simulink model "environment_simulation"  (R2022a)
settings: Solver=ode15s  StartTime=0.0  StopTime=42000  RelTol=1e-3
InitFcn:
  | global LOData LOModelData gprMdlLP_machine1 gprMdlLP_machine2 gprMdlLP_machine3 gprMdlLP_machine4 gprMdlLP_machine5 significance SteadyState explore explore_signal
  | load load_opt_multiple_init.mat
undefined symbols (not defined in the file or in its folder): sigbuilder_block
libraries: slpidlib x12, simulink x10
(part 1 of 2)
settings Model: Creator=Memo Mer  LastModifiedBy=busesibelkorkmaz
settings SolverCC: AlgebraicLoopSolver=TrustRegion
settings DebuggingCC: UnconnectedInputMsg=warning  UnconnectedOutputMsg=warning  UnconnectedLineMsg=warning  SFMachineParentedDataDiag=warning
settings RTWCC: DLArmComputeVersion=19.05

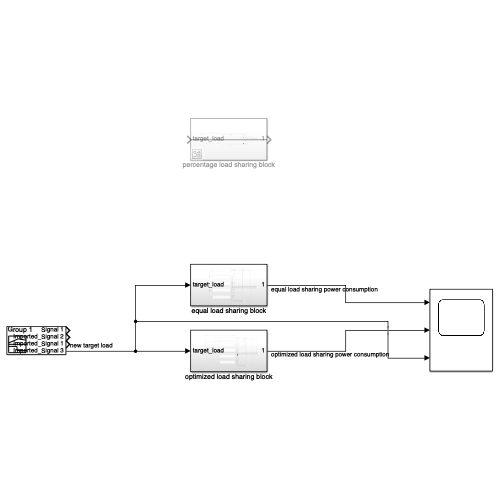
[thumbnail: Simulink's stored preview of the top-level diagram]
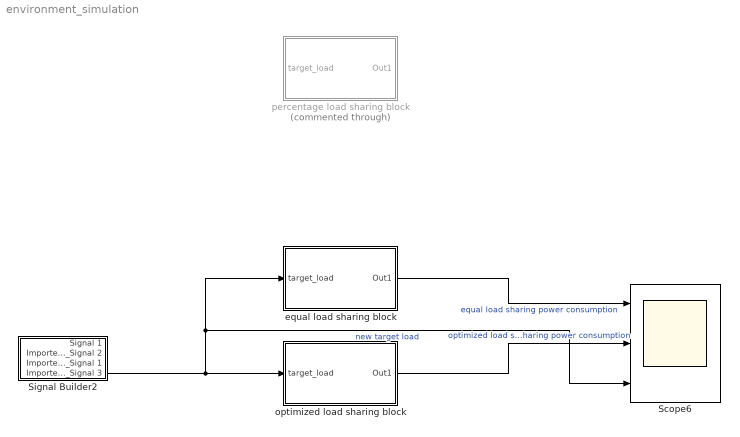
== system environment_simulation ==
  Scope6 : Scope  NumInputPorts=3
  Signal Builder2 : Subsystem  Tag=STV Subsys  LoadFcn=sigbuilder_block('load');  StartFcn=sigbuilder_block('start');  StopFcn=sigbuilder_block('stop');  ClipboardFcn=sigbuilder_block('clipboard');  mask(Sigbuilder block){tuvar=[0:10]}
      mask help: Simulink:masks:SigbuilderBlock_MD
      mask init:
      | if ~strcmp(get_param(bdroot(gcbh),'SimulationStatus'),'stopped') tuvar = sigbuilder_block('maskInit'); end
      settings: CopyFcn=sigbuilder_block('copy');  DeleteFcn=sigbuilder_block('delete');  ModelCloseFcn=sigbuilder_block('modelClose');  PreSaveFcn=sigbuilder_block('preSave');  PauseFcn=sigbuilder_block('pause');  ContinueFcn=sigbuilder_block('continue');  NameChangeFcn=sigbuilder_block('namechange');  OpenFcn=sigbuilder_block('open',[13 58 890 740 ]);  CloseFcn=sigbuilder_block('close');
      mask Display: plot(0, 0, 100, 100,[2, 2, 32, 32, 2], [68, 8, 8, 68, 68],[32, 2], [38, 38], [32, 19, 2],[53, 60, 44], [32, 17, 17, 2],[16, 16, 31, 31]);txt = getActiveGroup(gcbh);text(2, 100, txt,'verticalAlignment', 'top');
  equal load sharing block : Subsystem  Tag=equal load sharing
  optimized load sharing block : Subsystem  Tag=equal load sharing
  percentage load sharing block : Subsystem  Tag=equal load sharing  Commented=through
  wires:
  Signal Builder2/4(Imported_Signal 3) -> Scope6/3, equal load sharing block/1(target_load), optimized load sharing block/1(target_load)  "new target load"
  optimized load sharing block/1(Out1) -> Scope6/2  "optimized load sharing power consumption"
  equal load sharing block/1(Out1) -> Scope6/1  "equal load sharing power consumption"

== system environment_simulation/Signal Builder2 ==
  Demux : Demux  Tag=STV Demux
      settings: DisplayOption=none
  FromWs : FromWorkspace  Tag=STV FromWs  VariableName=tuvar
      SigBuilderData=|
      | common.afterFinalStr = 'Extrapolate'
      | common.sampleTime = '0'
      | dataSet.timeRange = [0 42000]
      | dataSet.name = 'Group 1'
      | sbobj.Groups.Name = 'Group 1'
      | sbobj.Groups.Signals(1).Name = 'Signal 1'
      | sbobj.Groups.Signals(1).XData = [0 200 200 400 400 600 600 800 800 1000 1000 1200 1200 1400 1400 1600 1600 1800 1800 2000 2000 2200 2200 2400 2400 2600 2620 4200 42000]
      | sbobj.Groups.Signals(1).YData = [0 0 -3.904416471 -3.904416471 -9.753929308 -9.753929308 -21.01201906 -21.01201906 -32.66837352 -32.66837352 3.755067207 3.755067207 7.595476851 7.5955 23.08157315 23.0816 19.1700448 19.1700448 28.04921414 28.04921414 27.99587512 27.99587512 28.33368893 28.3337 20.90889695 20.90889695 28.67505867 28.5998696218 28.5998696218]
      | sbobj.Groups.Signals(2).Name = 'Imported_Signal 2'
      | sbobj.Groups.Signals(2).XData = [0 200 200 400 400 600 600 800 800 1000 1000 1200 1200 1400 1400 1600 1600 1800 1800 2000 2000 2200 2200 2400 2400 2600 2600 2800 2800 3000 3000 3200 3200 3400 3400 3600 3600 3800 3800 4000 4000 42000]
      | sbobj.Groups.Signals(2).YData = [67.81523362 67.81523362 63.91081715 63.91081715 58.06130431 58.06130431 46.80321456 46.80321456 35.1468601 35.1468601 71.57030083 71.57030083 75.41071047 75.41071047 90.89680677 90.89680677 86.98527842 86.98527842 95.86444776 95.86444776 95.81110874 95.81110874 96.14892255 96.14892255 96.49029229 96.49029229 88.72413057 88.72413057 75.49249697 75.49249697 54.52670507 54.52670507 32.00341369 32.00341369 38.94815446 38.94815446 22.26370812 22.26370812 22.9855629 22.9855629 11.35409999 11.35409999]
      | sbobj.Groups.Signals(3).Name = 'Imported_Signal 1'
      | sbobj.Groups.Signals(3).XData = [0 200 200 400 400 600 600 800 800 1000 1000 1200 1200 1400 1400 1600 1600 1800 1800 2000 2000 2200 2200 2400 2400 2600 2600 2800 2800 3000 3000 3200 3200 3400 3400 3600 3600 3800 3800 4000 4000 42000]
      | sbobj.Groups.Signals(3).YData = [2130.75464 2130.75464 2008.077875 2008.077875 1824.286181 1824.286181 1470.557001 1470.557001 1104.314344 1104.314344 2248.738852 2248.738852 2369.404523 2369.404523 2855.977669 2855.977669 2733.077448 2733.077448 3012.060949 3012.060949 3010.385037 3010.385037 3020.999147 3020.999147 3031.724984 3031.724984 2787.712183 2787.712183 2371.974255 2371.974255 1713.229073 1713.229073 1005.547258 1005.547258 1223.751013 1223.751013 699.5257091 699.5257091 722.2063863 722.2063863 356.7458217 356.7458217]
      | sbobj.Groups.Signals(4).Name = 'Imported_Signal 3'
      | sbobj.Groups.Signals(4).XData = [0 1000 1000 2000 2000 3000 3000 4000 4000 5000 5000 6000 6000 7000 7000 8000 8000 9000 9000 10000 10000 11000 11000 12000 12000 13000 13000 14000 14000 15000 15000 16000 16000 17000 17000 18000 18000 19000 19000 20000 20000 21000 21000 22000 22000 23000 23000 24000 24000 25000 25000 26000 26000 27000 27000 28000 28000 29000 29000 30000 30000 31000 31000 32000 32000 33000 33000 34000 34000 35000 35000 36000 36000 37000 37000 38000 38000 39000 39000 40000 40000 41000 41000 42000]
      | sbobj.Groups.Signals(4).YData = [2130.75464 2130.75464 2008.077875 2008.077875 1824.286181 1824.286181 1470.557001 1470.557001 1104.314344 1104.314344 2248.738852 2248.738852 2369.404523 2369.404523 2855.977669 2855.977669 2733.077448 2733.077448 3012.060949 3012.060949 3010.385037 3010.385037 3020.999147 3020.999147 3031.724984 3031.724984 2787.712183 2787.712183 2371.974255 2371.974255 1713.229073 1713.229073 1005.547258 1005.547258 1223.751013 1223.751013 699.5257091 699.5257091 722.2063863 722.2063863 356.7458217 356.7458217 391.7165208 391.7165208 658.6334542 658.6334542 292.2790697 292.2790697 132.7322379 132.7322379 473.2775761 473.2775761 240.7727045 240.7727045 654.2760827 654.2760827 1287.435673 1287.435673 1396.258232 1396.258232 2089.862385 2089.862385 1516.812175 1516.812175 2198.573217 2198.573217 1028.8983 1028.8983 2684.81118 2684.81118 601.7641704 601.7641704 2757.210582 2757.210582 2915.081502 2915.081502 2281.363274 2281.363274 1670.549178 1670.549178 1876.909821 1876.909821 1425.53083 1425.53083]
      | sbobj.Groups.TimeRange = [0 42000]
  Signal 1 : Outport  Tag=STV Outport
  Imported_Signal 2 : Outport  Tag=STV Outport  Port=2
  Imported_Signal 1 : Outport  Tag=STV Outport  Port=3
  Imported_Signal 3 : Outport  Tag=STV Outport  Port=4
  wires:
  Demux/1 -> Signal 1/1
  FromWs/1 -> Demux/1
  Demux/2 -> Imported_Signal 2/1
  Demux/3 -> Imported_Signal 1/1
  Demux/4 -> Imported_Signal 3/1

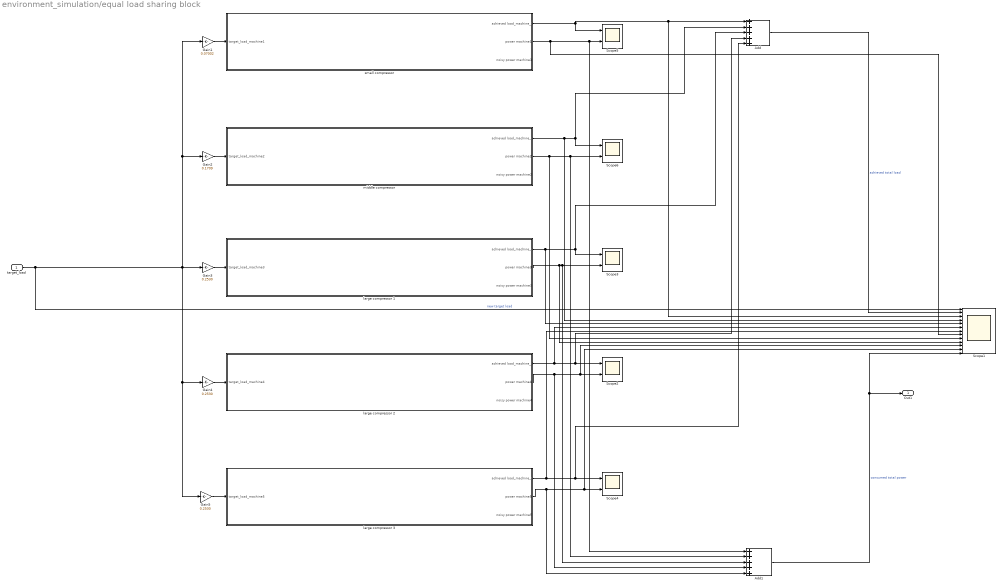
== system environment_simulation/equal load sharing block ==
  target_load : Inport
  Add : Sum  Inputs=+++++
  Add1 : Sum  Inputs=+++++
  Gain1 : Gain  Gain=0.07002
  Gain2 : Gain  Gain=0.1709
  Gain3 : Gain  Gain=0.2530
  Gain4 : Gain  Gain=0.2530
  Gain5 : Gain  Gain=0.2530
  Scope1 : Scope  NumInputPorts=13
  Scope{2..6} (5 alike) : Scope  NumInputPorts=2
  large compressor 1 : Subsystem
  large compressor 2 : Subsystem
  large compressor 3 : Subsystem
  middle compressor : Subsystem
  small compressor : Subsystem
  Out1 : Outport
  wires:
  Add/1 -> Scope1/2  "achieved total load"
  large compressor 1/1(achieved load_machine_3) -> Scope1/5, Scope3/1, Add/3
  middle compressor/1(achieved load_machine_2) -> Scope1/4, Scope6/1, Add/2
  small compressor/2(power machine1) -> Scope1/8, Add1/1, Scope5/2
  large compressor 3/1(achieved load_machine_5) -> Scope1/7, Add/5, Scope4/1
  middle compressor/2(power machine2) -> Scope1/9, Add1/2, Scope6/2
  large compressor 3/2(power machine5) -> Add1/5, Scope1/12, Scope4/2
  large compressor 2/2(power machine4) -> Add1/4, Scope1/11, Scope2/2
  target_load/1 -> Gain1/1, Gain2/1, Gain5/1, Gain4/1, Gain3/1, Scope1/1  "new target load"
  small compressor/1(achieved load_machine_1) -> Scope5/1, Scope1/3, Add/1
  Add1/1 -> Out1/1, Scope1/13  "consumed total power"
  large compressor 1/2(power machine3) -> Scope1/10, Add1/3, Scope3/2
  large compressor 2/1(achieved load_machine_4) -> Scope1/6, Add/4, Scope2/1
  Gain1/1 -> small compressor/1(target_load_machine1)
  Gain2/1 -> middle compressor/1(target_load_machine2)
  Gain3/1 -> large compressor 1/1(target_load_machine3)
  Gain4/1 -> large compressor 2/1(target_load_machine4)
  Gain5/1 -> large compressor 3/1(target_load_machine5)

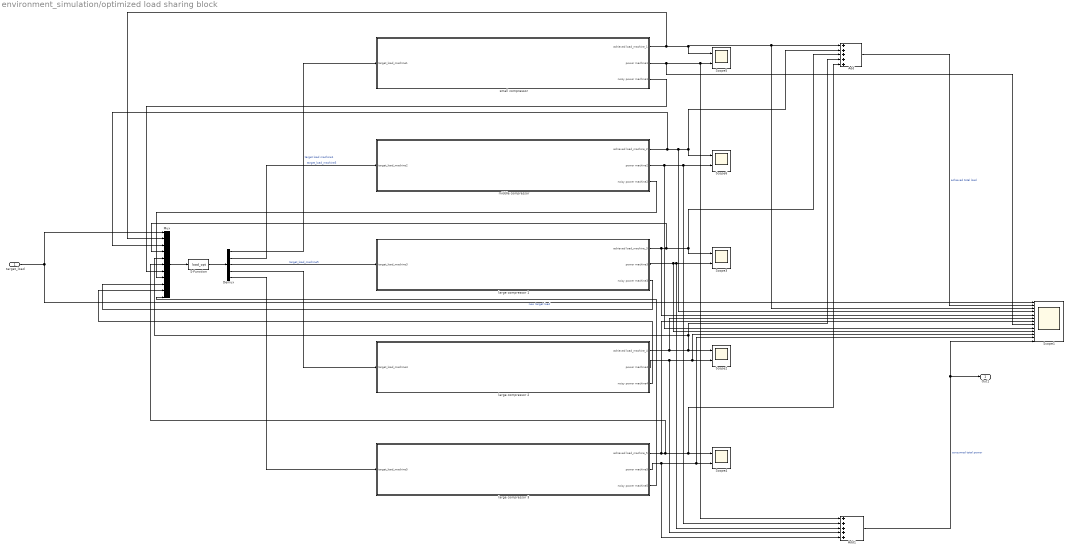
== system environment_simulation/optimized load sharing block ==
  target_load : Inport
  Add : Sum  Inputs=+++++
  Add1 : Sum  Inputs=+++++
  Demux : Demux  Outputs=5
  Mux : Mux  Inputs=11
  S-Function : S-Function  FunctionName=load_opt  Parameters=[],[]  SFunctionDeploymentMode=off  EnableBusSupport=off
  Scope1 : Scope  NumInputPorts=13
  Scope{2..6} (5 alike) : Scope  NumInputPorts=2
  large compressor 1 : Subsystem
  large compressor 2 : Subsystem
  large compressor 3 : Subsystem
  middle compressor : Subsystem
  small compressor : Subsystem
  Out1 : Outport
  wires:
  Add/1 -> Scope1/2  "achieved total load"
  Add1/1 -> Out1/1, Scope1/13  "consumed total power"
  Mux/1 -> S-Function/1
  target_load/1 -> Mux/1, Scope1/1  "new target load"
  S-Function/1 -> Demux/1
  large compressor 1/1(achieved load_machine_3) -> Scope1/5, Mux/4, Scope3/1, Add/3
  large compressor 3/1(achieved load_machine_5) -> Scope1/7, Mux/6, Add/5, Scope4/1
  large compressor 3/2(power machine5) -> Add1/5, Scope1/12, Scope4/2
  middle compressor/1(achieved load_machine_2) -> Scope1/4, Scope6/1, Add/2, Mux/3
  middle compressor/2(power machine2) -> Scope1/9, Add1/2, Scope6/2
  small compressor/2(power machine1) -> Scope1/8, Add1/1, Scope5/2
  Demux/1 -> small compressor/1(target_load_machine1)  "target load machine1"
  Demux/2 -> middle compressor/1(target_load_machine2)  "target_load_machine5"
  Demux/3 -> large compressor 1/1(target_load_machine3)  "target_load_machine5"
  Demux/4 -> large compressor 2/1(target_load_machine4)
  Demux/5 -> large compressor 3/1(target_load_machine5)
  large compressor 3/3(noisy power machine5) -> Mux/11
  large compressor 2/3(noisy power machine4) -> Mux/10
  middle compressor/3(noisy power machine2) -> Mux/8
  large compressor 1/3(noisy power machine3) -> Mux/9
  small compressor/3(noisy power machine1) -> Mux/7
  small compressor/1(achieved load_machine_1) -> Scope5/1, Scope1/3, Add/1, Mux/2
  large compressor 1/2(power machine3) -> Scope1/10, Add1/3, Scope3/2
  large compressor 2/1(achieved load_machine_4) -> Scope1/6, Add/4, Mux/5, Scope2/1
  large compressor 2/2(power machine4) -> Add1/4, Scope1/11, Scope2/2

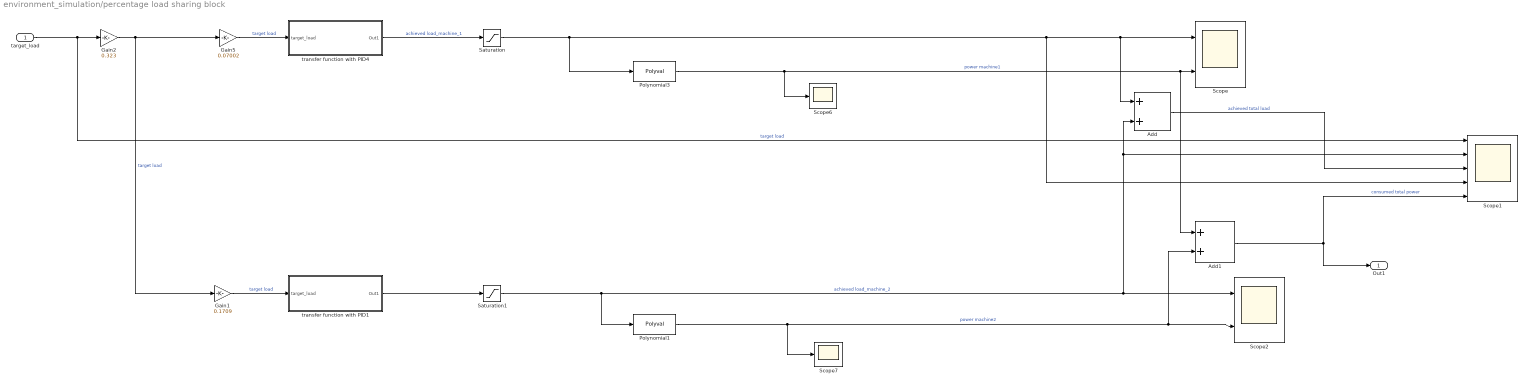
== system environment_simulation/percentage load sharing block ==
  target_load : Inport
  Add : Sum
  Add1 : Sum
  Gain1 : Gain  Gain=0.1709
  Gain2 : Gain  Gain=0.323
  Gain5 : Gain  Gain=0.07002
  Polynomial1 : Polyval  Coefs=[-1.42718017e-08 1.87477980e-05 -8.28649653e-03 1.88469092 -2.19952823]
  Polynomial3 : Polyval  Coefs=[-9e-08 4e-05 -0.0052 0.7765 15.661]
  Saturation : Saturate  UpperLimit=220  LowerLimit=56
  Saturation1 : Saturate  UpperLimit=537  LowerLimit=237
  Scope : Scope  NumInputPorts=2
  Scope1 : Scope  NumInputPorts=5
  Scope2 : Scope  NumInputPorts=2
  Scope6 : Scope
  Scope7 : Scope
  transfer function with PID1 : Subsystem
  transfer function with PID4 : Subsystem
  Out1 : Outport
  wires:
  Polynomial3/1 -> Scope6/1, Scope/2, Add1/1  "power machine1"
  transfer function with PID4/1(Out1) -> Saturation/1  "achieved load_machine_1"
  target_load/1 -> Gain2/1, Scope1/1  "target load"
  Saturation1/1 -> Polynomial1/1, Scope2/1, Add/2, Scope1/2  "achieved load_machine_2"
  transfer function with PID1/1(Out1) -> Saturation1/1
  Add/1 -> Scope1/3  "achieved total load"
  Add1/1 -> Scope1/5, Out1/1  "consumed total power"
  Polynomial1/1 -> Scope7/1, Scope2/2, Add1/2  "power machine2"
  Saturation/1 -> Polynomial3/1, Add/1, Scope/1, Scope1/4
  Gain5/1 -> transfer function with PID4/1(target_load)  "target load"
  Gain1/1 -> transfer function with PID1/1(target_load)  "target load"
  Gain2/1 -> Gain1/1, Gain5/1  "target load"

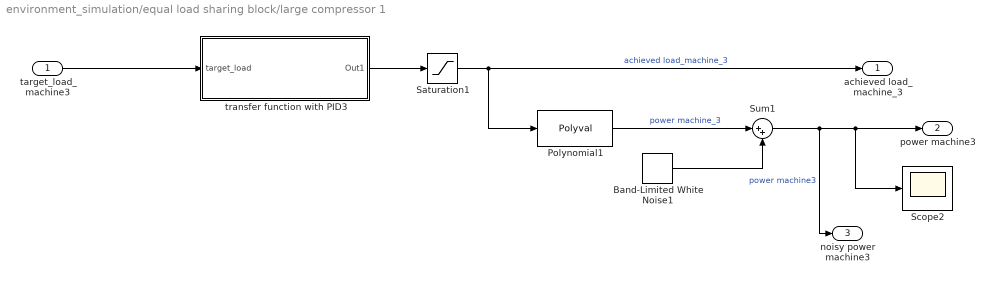
== system environment_simulation/equal load sharing block/large compressor 1 ==
  target_load_machine3 : Inport
  Band-Limited White Noise1 : simulink/Sources/Band-Limited White Noise  Cov=[0.1]  Ts=5  seed=[23341]
  Polynomial1 : Polyval  Coefs="[-1.53490519e-09  2.28838030e-06 -9.59520873e-04 6.18821903e-01 7.51758182e+01]"
  Saturation1 : Saturate  UpperLimit=795  LowerLimit=194
  Scope2 : Scope
  Sum1 : Sum  Inputs=|++
  transfer function with PID3 : Subsystem
  achieved load_machine_3 : Outport
  power machine3 : Outport  Port=2
  noisy power machine3 : Outport  Port=3
  wires:
  Polynomial1/1 -> Sum1/1  "power machine_3"
  target_load_machine3/1 -> transfer function with PID3/1(target_load)
  transfer function with PID3/1(Out1) -> Saturation1/1
  Band-Limited White Noise1/1 -> Sum1/2
  Saturation1/1 -> achieved load_machine_3/1, Polynomial1/1  "achieved load_machine_3"
  Sum1/1 -> noisy power machine3/1, power machine3/1, Scope2/1  "power machine3"

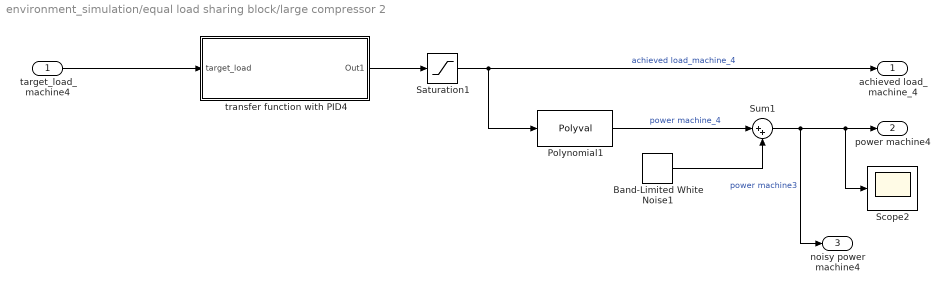
== system environment_simulation/equal load sharing block/large compressor 2 ==
  target_load_machine4 : Inport
  Band-Limited White Noise1 : simulink/Sources/Band-Limited White Noise  Cov=[0.1]  Ts=5  seed=[23341]
  Polynomial1 : Polyval  Coefs="[-1.53490519e-09  2.28838030e-06 -9.59520873e-04 6.18821903e-01 7.51758182e+01]"
  Saturation1 : Saturate  UpperLimit=795  LowerLimit=194
  Scope2 : Scope
  Sum1 : Sum  Inputs=|++
  transfer function with PID4 : Subsystem
  achieved load_machine_4 : Outport
  power machine4 : Outport  Port=2
  noisy power machine4 : Outport  Port=3
  wires:
  Polynomial1/1 -> Sum1/1  "power machine_4"
  Sum1/1 -> power machine4/1, Scope2/1, noisy power machine4/1  "power machine3"
  target_load_machine4/1 -> transfer function with PID4/1(target_load)
  transfer function with PID4/1(Out1) -> Saturation1/1
  Band-Limited White Noise1/1 -> Sum1/2
  Saturation1/1 -> achieved load_machine_4/1, Polynomial1/1  "achieved load_machine_4"

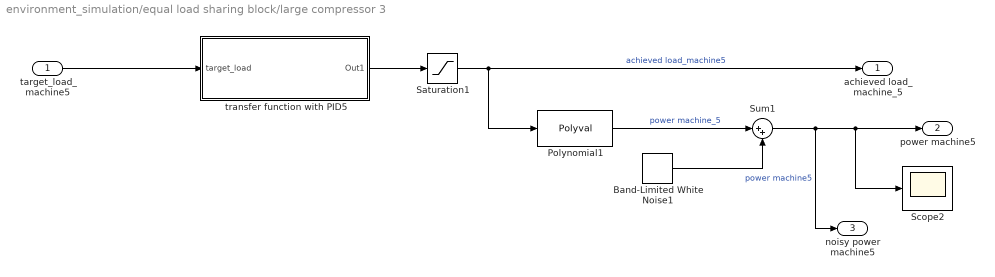
== system environment_simulation/equal load sharing block/large compressor 3 ==
  target_load_machine5 : Inport
  Band-Limited White Noise1 : simulink/Sources/Band-Limited White Noise  Cov=[0.1]  Ts=5  seed=[23341]
  Polynomial1 : Polyval  Coefs="[-1.53490519e-09  2.28838030e-06 -9.59520873e-04 6.18821903e-01 7.51758182e+01]"
  Saturation1 : Saturate  UpperLimit=795  LowerLimit=194
  Scope2 : Scope
  Sum1 : Sum  Inputs=|++
  transfer function with PID5 : Subsystem
  achieved load_machine_5 : Outport
  power machine5 : Outport  Port=2
  noisy power machine5 : Outport  Port=3
  wires:
  Polynomial1/1 -> Sum1/1  "power machine_5"
  target_load_machine5/1 -> transfer function with PID5/1(target_load)
  transfer function with PID5/1(Out1) -> Saturation1/1
  Band-Limited White Noise1/1 -> Sum1/2
  Saturation1/1 -> achieved load_machine_5/1, Polynomial1/1  "achieved load_machine5"
  Sum1/1 -> power machine5/1, Scope2/1, noisy power machine5/1  "power machine5"

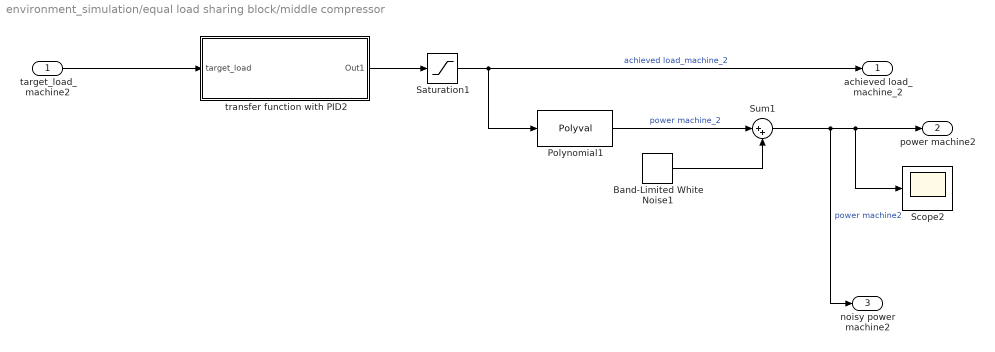
== system environment_simulation/equal load sharing block/middle compressor ==
  target_load_machine2 : Inport
  Band-Limited White Noise1 : simulink/Sources/Band-Limited White Noise  Cov=[0.1]  Ts=5  seed=[23341]
  Polynomial1 : Polyval  Coefs=[-1.42718017e-08 1.87477980e-05 -8.28649653e-03 1.88469092 -2.19952823]
  Saturation1 : Saturate  UpperLimit=537  LowerLimit=237
  Scope2 : Scope
  Sum1 : Sum  Inputs=|++
  transfer function with PID2 : Subsystem
  achieved load_machine_2 : Outport
  power machine2 : Outport  Port=2
  noisy power machine2 : Outport  Port=3
  wires:
  Polynomial1/1 -> Sum1/1  "power machine_2"
  target_load_machine2/1 -> transfer function with PID2/1(target_load)
  transfer function with PID2/1(Out1) -> Saturation1/1
  Band-Limited White Noise1/1 -> Sum1/2
  Saturation1/1 -> achieved load_machine_2/1, Polynomial1/1  "achieved load_machine_2"
  Sum1/1 -> noisy power machine2/1, power machine2/1, Scope2/1  "power machine2"

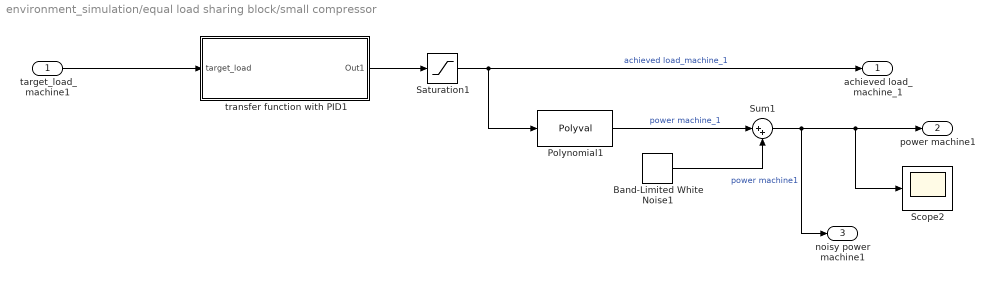
== system environment_simulation/equal load sharing block/small compressor ==
  target_load_machine1 : Inport
  Band-Limited White Noise1 : simulink/Sources/Band-Limited White Noise  Cov=[0.1]  Ts=5  seed=[23341]
  Polynomial1 : Polyval  Coefs=[-9e-08 4e-05 -0.0052 0.7765 15.661]
  Saturation1 : Saturate  UpperLimit=220  LowerLimit=56
  Scope2 : Scope
  Sum1 : Sum  Inputs=|++
  transfer function with PID1 : Subsystem
  achieved load_machine_1 : Outport
  power machine1 : Outport  Port=2
  noisy power machine1 : Outport  Port=3
  wires:
  Polynomial1/1 -> Sum1/1  "power machine_1"
  target_load_machine1/1 -> transfer function with PID1/1(target_load)
  transfer function with PID1/1(Out1) -> Saturation1/1
  Band-Limited White Noise1/1 -> Sum1/2
  Saturation1/1 -> achieved load_machine_1/1, Polynomial1/1  "achieved load_machine_1"
  Sum1/1 -> power machine1/1, Scope2/1, noisy power machine1/1  "power machine1"

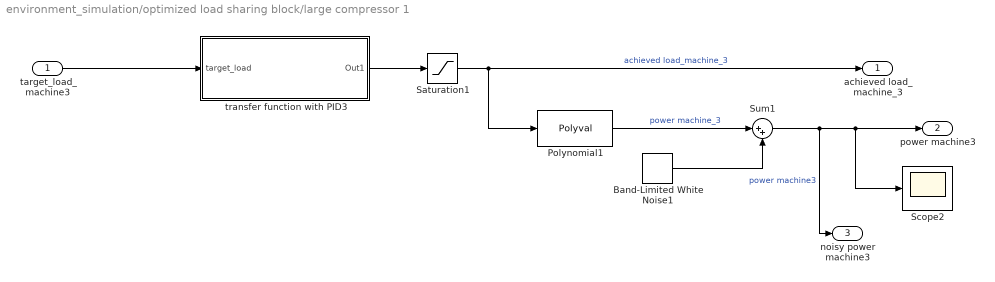
== system environment_simulation/optimized load sharing block/large compressor 1 ==
  target_load_machine3 : Inport
  Band-Limited White Noise1 : simulink/Sources/Band-Limited White Noise  Cov=[0.1]  Ts=5  seed=[23341]
  Polynomial1 : Polyval  Coefs="[-1.53490519e-09  2.28838030e-06 -9.59520873e-04 6.18821903e-01 7.51758182e+01]"
  Saturation1 : Saturate  UpperLimit=795  LowerLimit=194
  Scope2 : Scope
  Sum1 : Sum  Inputs=|++
  transfer function with PID3 : Subsystem
  achieved load_machine_3 : Outport
  power machine3 : Outport  Port=2
  noisy power machine3 : Outport  Port=3
  wires:
  Polynomial1/1 -> Sum1/1  "power machine_3"
  target_load_machine3/1 -> transfer function with PID3/1(target_load)
  transfer function with PID3/1(Out1) -> Saturation1/1
  Band-Limited White Noise1/1 -> Sum1/2
  Saturation1/1 -> achieved load_machine_3/1, Polynomial1/1  "achieved load_machine_3"
  Sum1/1 -> noisy power machine3/1, power machine3/1, Scope2/1  "power machine3"

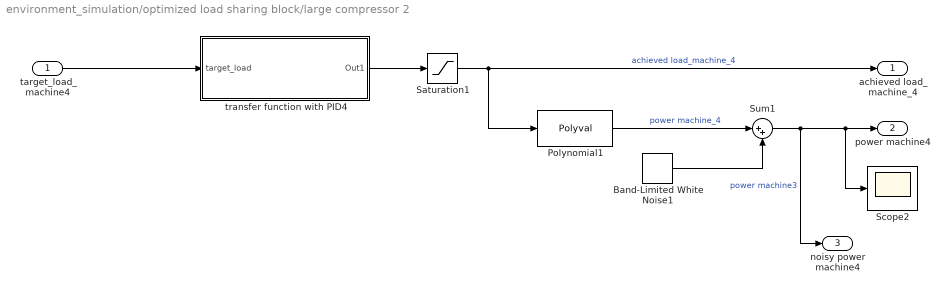
== system environment_simulation/optimized load sharing block/large compressor 2 ==
  target_load_machine4 : Inport
  Band-Limited White Noise1 : simulink/Sources/Band-Limited White Noise  Cov=[0.1]  Ts=5  seed=[23341]
  Polynomial1 : Polyval  Coefs="[-1.53490519e-09  2.28838030e-06 -9.59520873e-04 6.18821903e-01 7.51758182e+01]"
  Saturation1 : Saturate  UpperLimit=795  LowerLimit=194
  Scope2 : Scope
  Sum1 : Sum  Inputs=|++
  transfer function with PID4 : Subsystem
  achieved load_machine_4 : Outport
  power machine4 : Outport  Port=2
  noisy power machine4 : Outport  Port=3
  wires:
  Polynomial1/1 -> Sum1/1  "power machine_4"
  Sum1/1 -> power machine4/1, Scope2/1, noisy power machine4/1  "power machine3"
  target_load_machine4/1 -> transfer function with PID4/1(target_load)
  transfer function with PID4/1(Out1) -> Saturation1/1
  Band-Limited White Noise1/1 -> Sum1/2
  Saturation1/1 -> achieved load_machine_4/1, Polynomial1/1  "achieved load_machine_4"

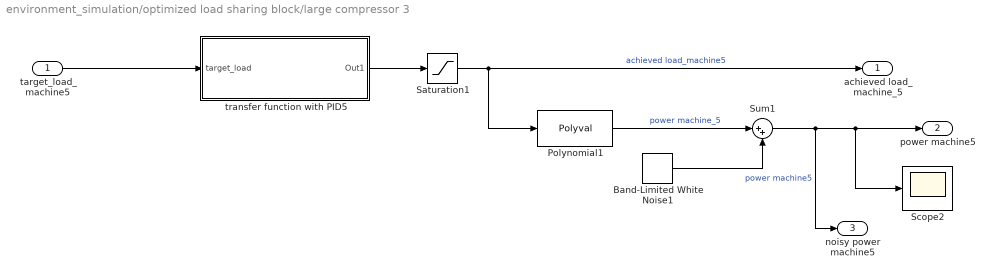
== system environment_simulation/optimized load sharing block/large compressor 3 ==
  target_load_machine5 : Inport
  Band-Limited White Noise1 : simulink/Sources/Band-Limited White Noise  Cov=[0.1]  Ts=5  seed=[23341]
  Polynomial1 : Polyval  Coefs="[-1.53490519e-09  2.28838030e-06 -9.59520873e-04 6.18821903e-01 7.51758182e+01]"
  Saturation1 : Saturate  UpperLimit=795  LowerLimit=194
  Scope2 : Scope
  Sum1 : Sum  Inputs=|++
  transfer function with PID5 : Subsystem
  achieved load_machine_5 : Outport
  power machine5 : Outport  Port=2
  noisy power machine5 : Outport  Port=3
  wires:
  Polynomial1/1 -> Sum1/1  "power machine_5"
  target_load_machine5/1 -> transfer function with PID5/1(target_load)
  transfer function with PID5/1(Out1) -> Saturation1/1
  Band-Limited White Noise1/1 -> Sum1/2
  Saturation1/1 -> achieved load_machine_5/1, Polynomial1/1  "achieved load_machine5"
  Sum1/1 -> power machine5/1, Scope2/1, noisy power machine5/1  "power machine5"

== system environment_simulation/optimized load sharing block/middle compressor ==
  target_load_machine2 : Inport
  Band-Limited White Noise1 : simulink/Sources/Band-Limited White Noise  Cov=[0.1]  Ts=5  seed=[23341]
  Polynomial1 : Polyval  Coefs=[-1.42718017e-08 1.87477980e-05 -8.28649653e-03 1.88469092 -2.19952823]
  Saturation1 : Saturate  UpperLimit=537  LowerLimit=237
  Scope2 : Scope
  Sum1 : Sum  Inputs=|++
  transfer function with PID2 : Subsystem
  achieved load_machine_2 : Outport
  power machine2 : Outport  Port=2
  noisy power machine2 : Outport  Port=3
  wires:
  Polynomial1/1 -> Sum1/1  "power machine_2"
  target_load_machine2/1 -> transfer function with PID2/1(target_load)
  transfer function with PID2/1(Out1) -> Saturation1/1
  Band-Limited White Noise1/1 -> Sum1/2
  Saturation1/1 -> achieved load_machine_2/1, Polynomial1/1  "achieved load_machine_2"
  Sum1/1 -> noisy power machine2/1, power machine2/1, Scope2/1  "power machine2"

== system environment_simulation/optimized load sharing block/small compressor ==
  target_load_machine1 : Inport
  Band-Limited White Noise1 : simulink/Sources/Band-Limited White Noise  Cov=[0.1]  Ts=5  seed=[23341]
  Polynomial1 : Polyval  Coefs=[-9e-08 4e-05 -0.0052 0.7765 15.661]
  Saturation1 : Saturate  UpperLimit=220  LowerLimit=56
  Scope2 : Scope
  Sum1 : Sum  Inputs=|++
  transfer function with PID1 : Subsystem
  achieved load_machine_1 : Outport
  power machine1 : Outport  Port=2
  noisy power machine1 : Outport  Port=3
  wires:
  Polynomial1/1 -> Sum1/1  "power machine_1"
  target_load_machine1/1 -> transfer function with PID1/1(target_load)
  transfer function with PID1/1(Out1) -> Saturation1/1
  Band-Limited White Noise1/1 -> Sum1/2
  Saturation1/1 -> achieved load_machine_1/1, Polynomial1/1  "achieved load_machine_1"
  Sum1/1 -> power machine1/1, Scope2/1, noisy power machine1/1  "power machine1"

== system environment_simulation/percentage load sharing block/transfer function with PID1 ==
  target_load : Inport
  GenSet_1_Dyn : TransferFcn  Denominator=[200 1]
  GenSet_1_Load_Ctrl : slpidlib/PID Controller (2DOF)  Controller=PID  Form=Parallel  TimeDomain=Continuous-time  UseExternalTs=off  SampleTime=-1  IntegratorMethod=Forward Euler  FilterMethod=Forward Euler  ControllerParametersSource=internal  P=100  I=10  UseKiTs=off  D=0  N=100  UseFilter=on  b=1  c=1  TunerSelectOption=Transfer Function Based (PID Tuner App)  InitialConditionSource=internal  InitialConditionForIntegrator=0  InitialConditionForFilter=0  DifferentiatorICPrevScaledInput=0  ExternalReset=none  TrackingMode=off  Kt=1  LimitOutput=off  SatLimitsSource=internal  UpperSaturationLimit=inf  LowerSaturationLimit=-inf  LinearizeAsGain=on  AntiWindupMode=none  Kb=1  POutMin=[]  POutMax=[]  IOutMin=[]  IOutMax=[]  DOutMin=[]  DOutMax=[]  NOutMin=[]  NOutMax=[]  bOutMin=[]  bOutMax=[]  cOutMin=[]  cOutMax=[]  SumOutMin=[]  SumOutMax=[]  SaturationOutMin=[]  SaturationOutMax=[]  PParamMin=[]  PParamMax=[]  IParamMin=[]  IParamMax=[]  DParamMin=[]  DParamMax=[]  NParamMin=[]  NParamMax=[]  bParamMin=[]  bParamMax=[]  cParamMin=[]  cParamMax=[]  KbParamMin=[]  KbParamMax=[]  KtParamMin=[]  KtParamMax=[]  KbOutMin=[]  KbOutMax=[]  KtOutMin=[]  KtOutMax=[]  IntegratorOutMin=[]  IntegratorOutMax=[]  FilterOutMin=[]  FilterOutMax=[]  SumI1OutMin=[]  SumI1OutMax=[]  SumI2OutMin=[]  SumI2OutMax=[]  SumI3OutMin=[]  SumI3OutMax=[]  SumI4OutMin=[]  SumI4OutMax=[]  SumDOutMin=[]  SumDOutMax=[]  Sum1OutMin=[]  Sum1OutMax=[]  Sum2OutMin=[]  Sum2OutMax=[]  Sum3OutMin=[]  Sum3OutMax=[]  DifferentiatorOutMin=[]  DifferentiatorOutMax=[]  FilterDiffOutCoefMin=[]  FilterDiffOutCoefMax=[]  ReciprocalOutMin=[]  ReciprocalOutMax=[]  SumDenOutMin=[]  SumDenOutMax=[]  SumNumOutMin=[]  SumNumOutMax=[]  DivideOutMin=[]  DivideOutMax=[]  UdiffTsProdOutMin=[]  UdiffTsProdOutMax=[]  NTsProdOutMin=[]  NTsProdOutMax=[]  UintegralTsProdOutMin=[]  UintegralTsProdOutMax=[]  UngainTsProdOutMin=[]  UngainTsProdOutMax=[]  IntegratorContinuousStateAttributes=''  IntegratorStateMustResolveToSignalObject=off  IntegratorRTWStateStorageClass=Auto  FilterContinuousStateAttributes=''  FilterStateMustResolveToSignalObject=off  FilterRTWStateStorageClass=Auto  ParallelPVariant=InternalParameters  IdealPVariant=Disabled  IVariant=InternalParameters  DVariant=InternalParameters  bVariant=InternalParameters  cVariant=InternalParameters  IntegratorVariant=Continuous  SatVariant=Disabled  AWVariant=Passthrough  PCopyVariant=Disabled  TRVariant=Disabled  FdbkBlocksVariant=Forward  IdealPFdbkVariant=Disabled  SatFdbkVariant=Disabled  DerivativeFilterVariant=ContFilter  NVariant=InternalParameters  NCopyVariant=Disabled  FilterICVariant=InternalICsFilter  IntegratorICVariant=InternalICs  ExternalResetVariant=Disabled  TRSumVariant=Passthrough  SumFdbkVariant=Disabled  SumVariant=Sum_PID  TsampFilterVariant=InternalTs  TsampNgainVariant=Passthrough  TsampIntegralVariant=Passthrough  ExternalSaturationOutDataTypeStr=Inherit: Same as second input
      settings: SourceProductBaseCode=SL
  Setpoint_Prefilter : TransferFcn  Denominator=[50 1]
  Out1 : Outport
  wires:
  GenSet_1_Load_Ctrl/1 -> GenSet_1_Dyn/1
  Setpoint_Prefilter/1 -> GenSet_1_Load_Ctrl/1
  target_load/1 -> Setpoint_Prefilter/1
  GenSet_1_Dyn/1 -> Out1/1, GenSet_1_Load_Ctrl/2

== system environment_simulation/percentage load sharing block/transfer function with PID4 ==
  target_load : Inport
  GenSet_1_Dyn : TransferFcn  Denominator=[200 1]
  GenSet_1_Load_Ctrl : slpidlib/PID Controller (2DOF)  Controller=PID  Form=Parallel  TimeDomain=Continuous-time  UseExternalTs=off  SampleTime=-1  IntegratorMethod=Forward Euler  FilterMethod=Forward Euler  ControllerParametersSource=internal  P=100  I=10  UseKiTs=off  D=0  N=100  UseFilter=on  b=1  c=1  TunerSelectOption=Transfer Function Based (PID Tuner App)  InitialConditionSource=internal  InitialConditionForIntegrator=0  InitialConditionForFilter=0  DifferentiatorICPrevScaledInput=0  ExternalReset=none  TrackingMode=off  Kt=1  LimitOutput=off  SatLimitsSource=internal  UpperSaturationLimit=inf  LowerSaturationLimit=-inf  LinearizeAsGain=on  AntiWindupMode=none  Kb=1  POutMin=[]  POutMax=[]  IOutMin=[]  IOutMax=[]  DOutMin=[]  DOutMax=[]  NOutMin=[]  NOutMax=[]  bOutMin=[]  bOutMax=[]  cOutMin=[]  cOutMax=[]  SumOutMin=[]  SumOutMax=[]  SaturationOutMin=[]  SaturationOutMax=[]  PParamMin=[]  PParamMax=[]  IParamMin=[]  IParamMax=[]  DParamMin=[]  DParamMax=[]  NParamMin=[]  NParamMax=[]  bParamMin=[]  bParamMax=[]  cParamMin=[]  cParamMax=[]  KbParamMin=[]  KbParamMax=[]  KtParamMin=[]  KtParamMax=[]  KbOutMin=[]  KbOutMax=[]  KtOutMin=[]  KtOutMax=[]  IntegratorOutMin=[]  IntegratorOutMax=[]  FilterOutMin=[]  FilterOutMax=[]  SumI1OutMin=[]  SumI1OutMax=[]  SumI2OutMin=[]  SumI2OutMax=[]  SumI3OutMin=[]  SumI3OutMax=[]  SumI4OutMin=[]  SumI4OutMax=[]  SumDOutMin=[]  SumDOutMax=[]  Sum1OutMin=[]  Sum1OutMax=[]  Sum2OutMin=[]  Sum2OutMax=[]  Sum3OutMin=[]  Sum3OutMax=[]  DifferentiatorOutMin=[]  DifferentiatorOutMax=[]  FilterDiffOutCoefMin=[]  FilterDiffOutCoefMax=[]  ReciprocalOutMin=[]  ReciprocalOutMax=[]  SumDenOutMin=[]  SumDenOutMax=[]  SumNumOutMin=[]  SumNumOutMax=[]  DivideOutMin=[]  DivideOutMax=[]  UdiffTsProdOutMin=[]  UdiffTsProdOutMax=[]  NTsProdOutMin=[]  NTsProdOutMax=[]  UintegralTsProdOutMin=[]  UintegralTsProdOutMax=[]  UngainTsProdOutMin=[]  UngainTsProdOutMax=[]  IntegratorContinuousStateAttributes=''  IntegratorStateMustResolveToSignalObject=off  IntegratorRTWStateStorageClass=Auto  FilterContinuousStateAttributes=''  FilterStateMustResolveToSignalObject=off  FilterRTWStateStorageClass=Auto  ParallelPVariant=InternalParameters  IdealPVariant=Disabled  IVariant=InternalParameters  DVariant=InternalParameters  bVariant=InternalParameters  cVariant=InternalParameters  IntegratorVariant=Continuous  SatVariant=Disabled  AWVariant=Passthrough  PCopyVariant=Disabled  TRVariant=Disabled  FdbkBlocksVariant=Forward  IdealPFdbkVariant=Disabled  SatFdbkVariant=Disabled  DerivativeFilterVariant=ContFilter  NVariant=InternalParameters  NCopyVariant=Disabled  FilterICVariant=InternalICsFilter  IntegratorICVariant=InternalICs  ExternalResetVariant=Disabled  TRSumVariant=Passthrough  SumFdbkVariant=Disabled  SumVariant=Sum_PID  TsampFilterVariant=InternalTs  TsampNgainVariant=Passthrough  TsampIntegralVariant=Passthrough  ExternalSaturationOutDataTypeStr=Inherit: Same as second input
      settings: SourceProductBaseCode=SL
  Setpoint_Prefilter : TransferFcn  Denominator=[50 1]
  Out1 : Outport
  wires:
  GenSet_1_Load_Ctrl/1 -> GenSet_1_Dyn/1
  Setpoint_Prefilter/1 -> GenSet_1_Load_Ctrl/1
  target_load/1 -> Setpoint_Prefilter/1
  GenSet_1_Dyn/1 -> Out1/1, GenSet_1_Load_Ctrl/2

== system environment_simulation/equal load sharing block/large compressor 1/transfer function with PID3 ==
  target_load : Inport
  GenSet_1_Dyn : TransferFcn  Denominator=[200 1]
  GenSet_1_Load_Ctrl : slpidlib/PID Controller (2DOF)  Controller=PID  Form=Parallel  TimeDomain=Continuous-time  UseExternalTs=off  SampleTime=-1  IntegratorMethod=Forward Euler  FilterMethod=Forward Euler  ControllerParametersSource=internal  P=100  I=10  UseKiTs=off  D=0  N=100  UseFilter=on  b=1  c=1  TunerSelectOption=Transfer Function Based (PID Tuner App)  InitialConditionSource=internal  InitialConditionForIntegrator=0  InitialConditionForFilter=0  DifferentiatorICPrevScaledInput=0  ExternalReset=none  TrackingMode=off  Kt=1  LimitOutput=off  SatLimitsSource=internal  UpperSaturationLimit=inf  LowerSaturationLimit=-inf  LinearizeAsGain=on  AntiWindupMode=none  Kb=1  POutMin=[]  POutMax=[]  IOutMin=[]  IOutMax=[]  DOutMin=[]  DOutMax=[]  NOutMin=[]  NOutMax=[]  bOutMin=[]  bOutMax=[]  cOutMin=[]  cOutMax=[]  SumOutMin=[]  SumOutMax=[]  SaturationOutMin=[]  SaturationOutMax=[]  PParamMin=[]  PParamMax=[]  IParamMin=[]  IParamMax=[]  DParamMin=[]  DParamMax=[]  NParamMin=[]  NParamMax=[]  bParamMin=[]  bParamMax=[]  cParamMin=[]  cParamMax=[]  KbParamMin=[]  KbParamMax=[]  KtParamMin=[]  KtParamMax=[]  KbOutMin=[]  KbOutMax=[]  KtOutMin=[]  KtOutMax=[]  IntegratorOutMin=[]  IntegratorOutMax=[]  FilterOutMin=[]  FilterOutMax=[]  SumI1OutMin=[]  SumI1OutMax=[]  SumI2OutMin=[]  SumI2OutMax=[]  SumI3OutMin=[]  SumI3OutMax=[]  SumI4OutMin=[]  SumI4OutMax=[]  SumDOutMin=[]  SumDOutMax=[]  Sum1OutMin=[]  Sum1OutMax=[]  Sum2OutMin=[]  Sum2OutMax=[]  Sum3OutMin=[]  Sum3OutMax=[]  DifferentiatorOutMin=[]  DifferentiatorOutMax=[]  FilterDiffOutCoefMin=[]  FilterDiffOutCoefMax=[]  ReciprocalOutMin=[]  ReciprocalOutMax=[]  SumDenOutMin=[]  SumDenOutMax=[]  SumNumOutMin=[]  SumNumOutMax=[]  DivideOutMin=[]  DivideOutMax=[]  UdiffTsProdOutMin=[]  UdiffTsProdOutMax=[]  NTsProdOutMin=[]  NTsProdOutMax=[]  UintegralTsProdOutMin=[]  UintegralTsProdOutMax=[]  UngainTsProdOutMin=[]  UngainTsProdOutMax=[]  IntegratorContinuousStateAttributes=''  IntegratorStateMustResolveToSignalObject=off  IntegratorRTWStateStorageClass=Auto  FilterContinuousStateAttributes=''  FilterStateMustResolveToSignalObject=off  FilterRTWStateStorageClass=Auto  ParallelPVariant=InternalParameters  IdealPVariant=Disabled  IVariant=InternalParameters  DVariant=InternalParameters  bVariant=InternalParameters  cVariant=InternalParameters  IntegratorVariant=Continuous  SatVariant=Disabled  AWVariant=Passthrough  PCopyVariant=Disabled  TRVariant=Disabled  FdbkBlocksVariant=Forward  IdealPFdbkVariant=Disabled  SatFdbkVariant=Disabled  DerivativeFilterVariant=ContFilter  NVariant=InternalParameters  NCopyVariant=Disabled  FilterICVariant=InternalICsFilter  IntegratorICVariant=InternalICs  ExternalResetVariant=Disabled  TRSumVariant=Passthrough  SumFdbkVariant=Disabled  SumVariant=Sum_PID  TsampFilterVariant=InternalTs  TsampNgainVariant=Passthrough  TsampIntegralVariant=Passthrough  ExternalSaturationOutDataTypeStr=Inherit: Same as second input
      settings: SourceProductBaseCode=SL
  Setpoint_Prefilter : TransferFcn  Denominator=[50 1]
  Out1 : Outport
  wires:
  GenSet_1_Load_Ctrl/1 -> GenSet_1_Dyn/1
  Setpoint_Prefilter/1 -> GenSet_1_Load_Ctrl/1
  target_load/1 -> Setpoint_Prefilter/1
  GenSet_1_Dyn/1 -> Out1/1, GenSet_1_Load_Ctrl/2

== system environment_simulation/equal load sharing block/large compressor 2/transfer function with PID4 ==
  target_load : Inport
  GenSet_1_Dyn : TransferFcn  Denominator=[200 1]
  GenSet_1_Load_Ctrl : slpidlib/PID Controller (2DOF)  Controller=PID  Form=Parallel  TimeDomain=Continuous-time  UseExternalTs=off  SampleTime=-1  IntegratorMethod=Forward Euler  FilterMethod=Forward Euler  ControllerParametersSource=internal  P=100  I=10  UseKiTs=off  D=0  N=100  UseFilter=on  b=1  c=1  TunerSelectOption=Transfer Function Based (PID Tuner App)  InitialConditionSource=internal  InitialConditionForIntegrator=0  InitialConditionForFilter=0  DifferentiatorICPrevScaledInput=0  ExternalReset=none  TrackingMode=off  Kt=1  LimitOutput=off  SatLimitsSource=internal  UpperSaturationLimit=inf  LowerSaturationLimit=-inf  LinearizeAsGain=on  AntiWindupMode=none  Kb=1  POutMin=[]  POutMax=[]  IOutMin=[]  IOutMax=[]  DOutMin=[]  DOutMax=[]  NOutMin=[]  NOutMax=[]  bOutMin=[]  bOutMax=[]  cOutMin=[]  cOutMax=[]  SumOutMin=[]  SumOutMax=[]  SaturationOutMin=[]  SaturationOutMax=[]  PParamMin=[]  PParamMax=[]  IParamMin=[]  IParamMax=[]  DParamMin=[]  DParamMax=[]  NParamMin=[]  NParamMax=[]  bParamMin=[]  bParamMax=[]  cParamMin=[]  cParamMax=[]  KbParamMin=[]  KbParamMax=[]  KtParamMin=[]  KtParamMax=[]  KbOutMin=[]  KbOutMax=[]  KtOutMin=[]  KtOutMax=[]  IntegratorOutMin=[]  IntegratorOutMax=[]  FilterOutMin=[]  FilterOutMax=[]  SumI1OutMin=[]  SumI1OutMax=[]  SumI2OutMin=[]  SumI2OutMax=[]  SumI3OutMin=[]  SumI3OutMax=[]  SumI4OutMin=[]  SumI4OutMax=[]  SumDOutMin=[]  SumDOutMax=[]  Sum1OutMin=[]  Sum1OutMax=[]  Sum2OutMin=[]  Sum2OutMax=[]  Sum3OutMin=[]  Sum3OutMax=[]  DifferentiatorOutMin=[]  DifferentiatorOutMax=[]  FilterDiffOutCoefMin=[]  FilterDiffOutCoefMax=[]  ReciprocalOutMin=[]  ReciprocalOutMax=[]  SumDenOutMin=[]  SumDenOutMax=[]  SumNumOutMin=[]  SumNumOutMax=[]  DivideOutMin=[]  DivideOutMax=[]  UdiffTsProdOutMin=[]  UdiffTsProdOutMax=[]  NTsProdOutMin=[]  NTsProdOutMax=[]  UintegralTsProdOutMin=[]  UintegralTsProdOutMax=[]  UngainTsProdOutMin=[]  UngainTsProdOutMax=[]  IntegratorContinuousStateAttributes=''  IntegratorStateMustResolveToSignalObject=off  IntegratorRTWStateStorageClass=Auto  FilterContinuousStateAttributes=''  FilterStateMustResolveToSignalObject=off  FilterRTWStateStorageClass=Auto  ParallelPVariant=InternalParameters  IdealPVariant=Disabled  IVariant=InternalParameters  DVariant=InternalParameters  bVariant=InternalParameters  cVariant=InternalParameters  IntegratorVariant=Continuous  SatVariant=Disabled  AWVariant=Passthrough  PCopyVariant=Disabled  TRVariant=Disabled  FdbkBlocksVariant=Forward  IdealPFdbkVariant=Disabled  SatFdbkVariant=Disabled  DerivativeFilterVariant=ContFilter  NVariant=InternalParameters  NCopyVariant=Disabled  FilterICVariant=InternalICsFilter  IntegratorICVariant=InternalICs  ExternalResetVariant=Disabled  TRSumVariant=Passthrough  SumFdbkVariant=Disabled  SumVariant=Sum_PID  TsampFilterVariant=InternalTs  TsampNgainVariant=Passthrough  TsampIntegralVariant=Passthrough  ExternalSaturationOutDataTypeStr=Inherit: Same as second input
      settings: SourceProductBaseCode=SL
  Setpoint_Prefilter : TransferFcn  Denominator=[50 1]
  Out1 : Outport
  wires:
  GenSet_1_Load_Ctrl/1 -> GenSet_1_Dyn/1
  Setpoint_Prefilter/1 -> GenSet_1_Load_Ctrl/1
  target_load/1 -> Setpoint_Prefilter/1
  GenSet_1_Dyn/1 -> Out1/1, GenSet_1_Load_Ctrl/2

== system environment_simulation/equal load sharing block/large compressor 3/transfer function with PID5 ==
  target_load : Inport
  GenSet_1_Dyn : TransferFcn  Denominator=[200 1]
  GenSet_1_Load_Ctrl : slpidlib/PID Controller (2DOF)  Controller=PID  Form=Parallel  TimeDomain=Continuous-time  UseExternalTs=off  SampleTime=-1  IntegratorMethod=Forward Euler  FilterMethod=Forward Euler  ControllerParametersSource=internal  P=100  I=10  UseKiTs=off  D=0  N=100  UseFilter=on  b=1  c=1  TunerSelectOption=Transfer Function Based (PID Tuner App)  InitialConditionSource=internal  InitialConditionForIntegrator=0  InitialConditionForFilter=0  DifferentiatorICPrevScaledInput=0  ExternalReset=none  TrackingMode=off  Kt=1  LimitOutput=off  SatLimitsSource=internal  UpperSaturationLimit=inf  LowerSaturationLimit=-inf  LinearizeAsGain=on  AntiWindupMode=none  Kb=1  POutMin=[]  POutMax=[]  IOutMin=[]  IOutMax=[]  DOutMin=[]  DOutMax=[]  NOutMin=[]  NOutMax=[]  bOutMin=[]  bOutMax=[]  cOutMin=[]  cOutMax=[]  SumOutMin=[]  SumOutMax=[]  SaturationOutMin=[]  SaturationOutMax=[]  PParamMin=[]  PParamMax=[]  IParamMin=[]  IParamMax=[]  DParamMin=[]  DParamMax=[]  NParamMin=[]  NParamMax=[]  bParamMin=[]  bParamMax=[]  cParamMin=[]  cParamMax=[]  KbParamMin=[]  KbParamMax=[]  KtParamMin=[]  KtParamMax=[]  KbOutMin=[]  KbOutMax=[]  KtOutMin=[]  KtOutMax=[]  IntegratorOutMin=[]  IntegratorOutMax=[]  FilterOutMin=[]  FilterOutMax=[]  SumI1OutMin=[]  SumI1OutMax=[]  SumI2OutMin=[]  SumI2OutMax=[]  SumI3OutMin=[]  SumI3OutMax=[]  SumI4OutMin=[]  SumI4OutMax=[]  SumDOutMin=[]  SumDOutMax=[]  Sum1OutMin=[]  Sum1OutMax=[]  Sum2OutMin=[]  Sum2OutMax=[]  Sum3OutMin=[]  Sum3OutMax=[]  DifferentiatorOutMin=[]  DifferentiatorOutMax=[]  FilterDiffOutCoefMin=[]  FilterDiffOutCoefMax=[]  ReciprocalOutMin=[]  ReciprocalOutMax=[]  SumDenOutMin=[]  SumDenOutMax=[]  SumNumOutMin=[]  SumNumOutMax=[]  DivideOutMin=[]  DivideOutMax=[]  UdiffTsProdOutMin=[]  UdiffTsProdOutMax=[]  NTsProdOutMin=[]  NTsProdOutMax=[]  UintegralTsProdOutMin=[]  UintegralTsProdOutMax=[]  UngainTsProdOutMin=[]  UngainTsProdOutMax=[]  IntegratorContinuousStateAttributes=''  IntegratorStateMustResolveToSignalObject=off  IntegratorRTWStateStorageClass=Auto  FilterContinuousStateAttributes=''  FilterStateMustResolveToSignalObject=off  FilterRTWStateStorageClass=Auto  ParallelPVariant=InternalParameters  IdealPVariant=Disabled  IVariant=InternalParameters  DVariant=InternalParameters  bVariant=InternalParameters  cVariant=InternalParameters  IntegratorVariant=Continuous  SatVariant=Disabled  AWVariant=Passthrough  PCopyVariant=Disabled  TRVariant=Disabled  FdbkBlocksVariant=Forward  IdealPFdbkVariant=Disabled  SatFdbkVariant=Disabled  DerivativeFilterVariant=ContFilter  NVariant=InternalParameters  NCopyVariant=Disabled  FilterICVariant=InternalICsFilter  IntegratorICVariant=InternalICs  ExternalResetVariant=Disabled  TRSumVariant=Passthrough  SumFdbkVariant=Disabled  SumVariant=Sum_PID  TsampFilterVariant=InternalTs  TsampNgainVariant=Passthrough  TsampIntegralVariant=Passthrough  ExternalSaturationOutDataTypeStr=Inherit: Same as second input
      settings: SourceProductBaseCode=SL
  Setpoint_Prefilter : TransferFcn  Denominator=[50 1]
  Out1 : Outport
  wires:
  GenSet_1_Load_Ctrl/1 -> GenSet_1_Dyn/1
  Setpoint_Prefilter/1 -> GenSet_1_Load_Ctrl/1
  target_load/1 -> Setpoint_Prefilter/1
  GenSet_1_Dyn/1 -> Out1/1, GenSet_1_Load_Ctrl/2

== system environment_simulation/equal load sharing block/middle compressor/transfer function with PID2 ==
  target_load : Inport
  GenSet_1_Dyn : TransferFcn  Denominator=[200 1]
  GenSet_1_Load_Ctrl : slpidlib/PID Controller (2DOF)  Controller=PID  Form=Parallel  TimeDomain=Continuous-time  UseExternalTs=off  SampleTime=-1  IntegratorMethod=Forward Euler  FilterMethod=Forward Euler  ControllerParametersSource=internal  P=100  I=10  UseKiTs=off  D=0  N=100  UseFilter=on  b=1  c=1  TunerSelectOption=Transfer Function Based (PID Tuner App)  InitialConditionSource=internal  InitialConditionForIntegrator=0  InitialConditionForFilter=0  DifferentiatorICPrevScaledInput=0  ExternalReset=none  TrackingMode=off  Kt=1  LimitOutput=off  SatLimitsSource=internal  UpperSaturationLimit=inf  LowerSaturationLimit=-inf  LinearizeAsGain=on  AntiWindupMode=none  Kb=1  POutMin=[]  POutMax=[]  IOutMin=[]  IOutMax=[]  DOutMin=[]  DOutMax=[]  NOutMin=[]  NOutMax=[]  bOutMin=[]  bOutMax=[]  cOutMin=[]  cOutMax=[]  SumOutMin=[]  SumOutMax=[]  SaturationOutMin=[]  SaturationOutMax=[]  PParamMin=[]  PParamMax=[]  IParamMin=[]  IParamMax=[]  DParamMin=[]  DParamMax=[]  NParamMin=[]  NParamMax=[]  bParamMin=[]  bParamMax=[]  cParamMin=[]  cParamMax=[]  KbParamMin=[]  KbParamMax=[]  KtParamMin=[]  KtParamMax=[]  KbOutMin=[]  KbOutMax=[]  KtOutMin=[]  KtOutMax=[]  IntegratorOutMin=[]  IntegratorOutMax=[]  FilterOutMin=[]  FilterOutMax=[]  SumI1OutMin=[]  SumI1OutMax=[]  SumI2OutMin=[]  SumI2OutMax=[]  SumI3OutMin=[]  SumI3OutMax=[]  SumI4OutMin=[]  SumI4OutMax=[]  SumDOutMin=[]  SumDOutMax=[]  Sum1OutMin=[]  Sum1OutMax=[]  Sum2OutMin=[]  Sum2OutMax=[]  Sum3OutMin=[]  Sum3OutMax=[]  DifferentiatorOutMin=[]  DifferentiatorOutMax=[]  FilterDiffOutCoefMin=[]  FilterDiffOutCoefMax=[]  ReciprocalOutMin=[]  ReciprocalOutMax=[]  SumDenOutMin=[]  SumDenOutMax=[]  SumNumOutMin=[]  SumNumOutMax=[]  DivideOutMin=[]  DivideOutMax=[]  UdiffTsProdOutMin=[]  UdiffTsProdOutMax=[]  NTsProdOutMin=[]  NTsProdOutMax=[]  UintegralTsProdOutMin=[]  UintegralTsProdOutMax=[]  UngainTsProdOutMin=[]  UngainTsProdOutMax=[]  IntegratorContinuousStateAttributes=''  IntegratorStateMustResolveToSignalObject=off  IntegratorRTWStateStorageClass=Auto  FilterContinuousStateAttributes=''  FilterStateMustResolveToSignalObject=off  FilterRTWStateStorageClass=Auto  ParallelPVariant=InternalParameters  IdealPVariant=Disabled  IVariant=InternalParameters  DVariant=InternalParameters  bVariant=InternalParameters  cVariant=InternalParameters  IntegratorVariant=Continuous  SatVariant=Disabled  AWVariant=Passthrough  PCopyVariant=Disabled  TRVariant=Disabled  FdbkBlocksVariant=Forward  IdealPFdbkVariant=Disabled  SatFdbkVariant=Disabled  DerivativeFilterVariant=ContFilter  NVariant=InternalParameters  NCopyVariant=Disabled  FilterICVariant=InternalICsFilter  IntegratorICVariant=InternalICs  ExternalResetVariant=Disabled  TRSumVariant=Passthrough  SumFdbkVariant=Disabled  SumVariant=Sum_PID  TsampFilterVariant=InternalTs  TsampNgainVariant=Passthrough  TsampIntegralVariant=Passthrough  ExternalSaturationOutDataTypeStr=Inherit: Same as second input
      settings: SourceProductBaseCode=SL
  Setpoint_Prefilter : TransferFcn  Denominator=[50 1]
  Out1 : Outport
  wires:
  GenSet_1_Load_Ctrl/1 -> GenSet_1_Dyn/1
  Setpoint_Prefilter/1 -> GenSet_1_Load_Ctrl/1
  target_load/1 -> Setpoint_Prefilter/1
  GenSet_1_Dyn/1 -> Out1/1, GenSet_1_Load_Ctrl/2

== system environment_simulation/equal load sharing block/small compressor/transfer function with PID1 ==
  target_load : Inport
  GenSet_1_Dyn : TransferFcn  Denominator=[200 1]
  GenSet_1_Load_Ctrl : slpidlib/PID Controller (2DOF)  Controller=PID  Form=Parallel  TimeDomain=Continuous-time  UseExternalTs=off  SampleTime=-1  IntegratorMethod=Forward Euler  FilterMethod=Forward Euler  ControllerParametersSource=internal  P=100  I=10  UseKiTs=off  D=0  N=100  UseFilter=on  b=1  c=1  TunerSelectOption=Transfer Function Based (PID Tuner App)  InitialConditionSource=internal  InitialConditionForIntegrator=0  InitialConditionForFilter=0  DifferentiatorICPrevScaledInput=0  ExternalReset=none  TrackingMode=off  Kt=1  LimitOutput=off  SatLimitsSource=internal  UpperSaturationLimit=inf  LowerSaturationLimit=-inf  LinearizeAsGain=on  AntiWindupMode=none  Kb=1  POutMin=[]  POutMax=[]  IOutMin=[]  IOutMax=[]  DOutMin=[]  DOutMax=[]  NOutMin=[]  NOutMax=[]  bOutMin=[]  bOutMax=[]  cOutMin=[]  cOutMax=[]  SumOutMin=[]  SumOutMax=[]  SaturationOutMin=[]  SaturationOutMax=[]  PParamMin=[]  PParamMax=[]  IParamMin=[]  IParamMax=[]  DParamMin=[]  DParamMax=[]  NParamMin=[]  NParamMax=[]  bParamMin=[]  bParamMax=[]  cParamMin=[]  cParamMax=[]  KbParamMin=[]  KbParamMax=[]  KtParamMin=[]  KtParamMax=[]  KbOutMin=[]  KbOutMax=[]  KtOutMin=[]  KtOutMax=[]  IntegratorOutMin=[]  IntegratorOutMax=[]  FilterOutMin=[]  FilterOutMax=[]  SumI1OutMin=[]  SumI1OutMax=[]  SumI2OutMin=[]  SumI2OutMax=[]  SumI3OutMin=[]  SumI3OutMax=[]  SumI4OutMin=[]  SumI4OutMax=[]  SumDOutMin=[]  SumDOutMax=[]  Sum1OutMin=[]  Sum1OutMax=[]  Sum2OutMin=[]  Sum2OutMax=[]  Sum3OutMin=[]  Sum3OutMax=[]  DifferentiatorOutMin=[]  DifferentiatorOutMax=[]  FilterDiffOutCoefMin=[]  FilterDiffOutCoefMax=[]  ReciprocalOutMin=[]  ReciprocalOutMax=[]  SumDenOutMin=[]  SumDenOutMax=[]  SumNumOutMin=[]  SumNumOutMax=[]  DivideOutMin=[]  DivideOutMax=[]  UdiffTsProdOutMin=[]  UdiffTsProdOutMax=[]  NTsProdOutMin=[]  NTsProdOutMax=[]  UintegralTsProdOutMin=[]  UintegralTsProdOutMax=[]  UngainTsProdOutMin=[]  UngainTsProdOutMax=[]  IntegratorContinuousStateAttributes=''  IntegratorStateMustResolveToSignalObject=off  IntegratorRTWStateStorageClass=Auto  FilterContinuousStateAttributes=''  FilterStateMustResolveToSignalObject=off  FilterRTWStateStorageClass=Auto  ParallelPVariant=InternalParameters  IdealPVariant=Disabled  IVariant=InternalParameters  DVariant=InternalParameters  bVariant=InternalParameters  cVariant=InternalParameters  IntegratorVariant=Continuous  SatVariant=Disabled  AWVariant=Passthrough  PCopyVariant=Disabled  TRVariant=Disabled  FdbkBlocksVariant=Forward  IdealPFdbkVariant=Disabled  SatFdbkVariant=Disabled  DerivativeFilterVariant=ContFilter  NVariant=InternalParameters  NCopyVariant=Disabled  FilterICVariant=InternalICsFilter  IntegratorICVariant=InternalICs  ExternalResetVariant=Disabled  TRSumVariant=Passthrough  SumFdbkVariant=Disabled  SumVariant=Sum_PID  TsampFilterVariant=InternalTs  TsampNgainVariant=Passthrough  TsampIntegralVariant=Passthrough  ExternalSaturationOutDataTypeStr=Inherit: Same as second input
      settings: SourceProductBaseCode=SL
  Setpoint_Prefilter : TransferFcn  Denominator=[50 1]
  Out1 : Outport
  wires:
  GenSet_1_Load_Ctrl/1 -> GenSet_1_Dyn/1
  Setpoint_Prefilter/1 -> GenSet_1_Load_Ctrl/1
  target_load/1 -> Setpoint_Prefilter/1
  GenSet_1_Dyn/1 -> Out1/1, GenSet_1_Load_Ctrl/2

== system environment_simulation/optimized load sharing block/large compressor 1/transfer function with PID3 ==
  target_load : Inport
  GenSet_1_Dyn : TransferFcn  Denominator=[200 1]
  GenSet_1_Load_Ctrl : slpidlib/PID Controller (2DOF)  Controller=PID  Form=Parallel  TimeDomain=Continuous-time  UseExternalTs=off  SampleTime=-1  IntegratorMethod=Forward Euler  FilterMethod=Forward Euler  ControllerParametersSource=internal  P=100  I=10  UseKiTs=off  D=0  N=100  UseFilter=on  b=1  c=1  TunerSelectOption=Transfer Function Based (PID Tuner App)  InitialConditionSource=internal  InitialConditionForIntegrator=0  InitialConditionForFilter=0  DifferentiatorICPrevScaledInput=0  ExternalReset=none  TrackingMode=off  Kt=1  LimitOutput=off  SatLimitsSource=internal  UpperSaturationLimit=inf  LowerSaturationLimit=-inf  LinearizeAsGain=on  AntiWindupMode=none  Kb=1  POutMin=[]  POutMax=[]  IOutMin=[]  IOutMax=[]  DOutMin=[]  DOutMax=[]  NOutMin=[]  NOutMax=[]  bOutMin=[]  bOutMax=[]  cOutMin=[]  cOutMax=[]  SumOutMin=[]  SumOutMax=[]  SaturationOutMin=[]  SaturationOutMax=[]  PParamMin=[]  PParamMax=[]  IParamMin=[]  IParamMax=[]  DParamMin=[]  DParamMax=[]  NParamMin=[]  NParamMax=[]  bParamMin=[]  bParamMax=[]  cParamMin=[]  cParamMax=[]  KbParamMin=[]  KbParamMax=[]  KtParamMin=[]  KtParamMax=[]  KbOutMin=[]  KbOutMax=[]  KtOutMin=[]  KtOutMax=[]  IntegratorOutMin=[]  IntegratorOutMax=[]  FilterOutMin=[]  FilterOutMax=[]  SumI1OutMin=[]  SumI1OutMax=[]  SumI2OutMin=[]  SumI2OutMax=[]  SumI3OutMin=[]  SumI3OutMax=[]  SumI4OutMin=[]  SumI4OutMax=[]  SumDOutMin=[]  SumDOutMax=[]  Sum1OutMin=[]  Sum1OutMax=[]  Sum2OutMin=[]  Sum2OutMax=[]  Sum3OutMin=[]  Sum3OutMax=[]  DifferentiatorOutMin=[]  DifferentiatorOutMax=[]  FilterDiffOutCoefMin=[]  FilterDiffOutCoefMax=[]  ReciprocalOutMin=[]  ReciprocalOutMax=[]  SumDenOutMin=[]  SumDenOutMax=[]  SumNumOutMin=[]  SumNumOutMax=[]  DivideOutMin=[]  DivideOutMax=[]  UdiffTsProdOutMin=[]  UdiffTsProdOutMax=[]  NTsProdOutMin=[]  NTsProdOutMax=[]  UintegralTsProdOutMin=[]  UintegralTsProdOutMax=[]  UngainTsProdOutMin=[]  UngainTsProdOutMax=[]  IntegratorContinuousStateAttributes=''  IntegratorStateMustResolveToSignalObject=off  IntegratorRTWStateStorageClass=Auto  FilterContinuousStateAttributes=''  FilterStateMustResolveToSignalObject=off  FilterRTWStateStorageClass=Auto  ParallelPVariant=InternalParameters  IdealPVariant=Disabled  IVariant=InternalParameters  DVariant=InternalParameters  bVariant=InternalParameters  cVariant=InternalParameters  IntegratorVariant=Continuous  SatVariant=Disabled  AWVariant=Passthrough  PCopyVariant=Disabled  TRVariant=Disabled  FdbkBlocksVariant=Forward  IdealPFdbkVariant=Disabled  SatFdbkVariant=Disabled  DerivativeFilterVariant=ContFilter  NVariant=InternalParameters  NCopyVariant=Disabled  FilterICVariant=InternalICsFilter  IntegratorICVariant=InternalICs  ExternalResetVariant=Disabled  TRSumVariant=Passthrough  SumFdbkVariant=Disabled  SumVariant=Sum_PID  TsampFilterVariant=InternalTs  TsampNgainVariant=Passthrough  TsampIntegralVariant=Passthrough  ExternalSaturationOutDataTypeStr=Inherit: Same as second input
      settings: SourceProductBaseCode=SL
  Setpoint_Prefilter : TransferFcn  Denominator=[50 1]
  Out1 : Outport
  wires:
  GenSet_1_Load_Ctrl/1 -> GenSet_1_Dyn/1
  Setpoint_Prefilter/1 -> GenSet_1_Load_Ctrl/1
  target_load/1 -> Setpoint_Prefilter/1
  GenSet_1_Dyn/1 -> Out1/1, GenSet_1_Load_Ctrl/2

== system environment_simulation/optimized load sharing block/large compressor 2/transfer function with PID4 ==
  target_load : Inport
  GenSet_1_Dyn : TransferFcn  Denominator=[200 1]
  GenSet_1_Load_Ctrl : slpidlib/PID Controller (2DOF)  Controller=PID  Form=Parallel  TimeDomain=Continuous-time  UseExternalTs=off  SampleTime=-1  IntegratorMethod=Forward Euler  FilterMethod=Forward Euler  ControllerParametersSource=internal  P=100  I=10  UseKiTs=off  D=0  N=100  UseFilter=on  b=1  c=1  TunerSelectOption=Transfer Function Based (PID Tuner App)  InitialConditionSource=internal  InitialConditionForIntegrator=0  InitialConditionForFilter=0  DifferentiatorICPrevScaledInput=0  ExternalReset=none  TrackingMode=off  Kt=1  LimitOutput=off  SatLimitsSource=internal  UpperSaturationLimit=inf  LowerSaturationLimit=-inf  LinearizeAsGain=on  AntiWindupMode=none  Kb=1  POutMin=[]  POutMax=[]  IOutMin=[]  IOutMax=[]  DOutMin=[]  DOutMax=[]  NOutMin=[]  NOutMax=[]  bOutMin=[]  bOutMax=[]  cOutMin=[]  cOutMax=[]  SumOutMin=[]  SumOutMax=[]  SaturationOutMin=[]  SaturationOutMax=[]  PParamMin=[]  PParamMax=[]  IParamMin=[]  IParamMax=[]  DParamMin=[]  DParamMax=[]  NParamMin=[]  NParamMax=[]  bParamMin=[]  bParamMax=[]  cParamMin=[]  cParamMax=[]  KbParamMin=[]  KbParamMax=[]  KtParamMin=[]  KtParamMax=[]  KbOutMin=[]  KbOutMax=[]  KtOutMin=[]  KtOutMax=[]  IntegratorOutMin=[]  IntegratorOutMax=[]  FilterOutMin=[]  FilterOutMax=[]  SumI1OutMin=[]  SumI1OutMax=[]  SumI2OutMin=[]  SumI2OutMax=[]  SumI3OutMin=[]  SumI3OutMax=[]  SumI4OutMin=[]  SumI4OutMax=[]  SumDOutMin=[]  SumDOutMax=[]  Sum1OutMin=[]  Sum1OutMax=[]  Sum2OutMin=[]  Sum2OutMax=[]  Sum3OutMin=[]  Sum3OutMax=[]  DifferentiatorOutMin=[]  DifferentiatorOutMax=[]  FilterDiffOutCoefMin=[]  FilterDiffOutCoefMax=[]  ReciprocalOutMin=[]  ReciprocalOutMax=[]  SumDenOutMin=[]  SumDenOutMax=[]  SumNumOutMin=[]  SumNumOutMax=[]  DivideOutMin=[]  DivideOutMax=[]  UdiffTsProdOutMin=[]  UdiffTsProdOutMax=[]  NTsProdOutMin=[]  NTsProdOutMax=[]  UintegralTsProdOutMin=[]  UintegralTsProdOutMax=[]  UngainTsProdOutMin=[]  UngainTsProdOutMax=[]  IntegratorContinuousStateAttributes=''  IntegratorStateMustResolveToSignalObject=off  IntegratorRTWStateStorageClass=Auto  FilterContinuousStateAttributes=''  FilterStateMustResolveToSignalObject=off  FilterRTWStateStorageClass=Auto  ParallelPVariant=InternalParameters  IdealPVariant=Disabled  IVariant=InternalParameters  DVariant=InternalParameters  bVariant=InternalParameters  cVariant=InternalParameters  IntegratorVariant=Continuous  SatVariant=Disabled  AWVariant=Passthrough  PCopyVariant=Disabled  TRVariant=Disabled  FdbkBlocksVariant=Forward  IdealPFdbkVariant=Disabled  SatFdbkVariant=Disabled  DerivativeFilterVariant=ContFilter  NVariant=InternalParameters  NCopyVariant=Disabled  FilterICVariant=InternalICsFilter  IntegratorICVariant=InternalICs  ExternalResetVariant=Disabled  TRSumVariant=Passthrough  SumFdbkVariant=Disabled  SumVariant=Sum_PID  TsampFilterVariant=InternalTs  TsampNgainVariant=Passthrough  TsampIntegralVariant=Passthrough  ExternalSaturationOutDataTypeStr=Inherit: Same as second input
      settings: SourceProductBaseCode=SL
  Setpoint_Prefilter : TransferFcn  Denominator=[50 1]
  Out1 : Outport
  wires:
  GenSet_1_Load_Ctrl/1 -> GenSet_1_Dyn/1
  Setpoint_Prefilter/1 -> GenSet_1_Load_Ctrl/1
  target_load/1 -> Setpoint_Prefilter/1
  GenSet_1_Dyn/1 -> Out1/1, GenSet_1_Load_Ctrl/2
